simulink model "ltslqgservo"  (Simulink 8.0)
settings: Solver=ode1  StartTime=0.0  StopTime=stoptime  FixedStep=(1/10000)  RelTol=1e-3
values from neighbouring files (symbols this model uses):
  Ahat = Ap-Bp*Kpmcv    [main (ADMIN-PC's conflicted copy 2013-10-01).m]    (also in main.m = Ap-Bp*Kplqg)
  Ahat1 = Ayaw-Byaw*Kymcv    [main (ADMIN-PC's conflicted copy 2013-10-01).m]    (also in main.m = Ayaw-Byaw*Kylqg)
  Bhat = [Bp Gp]    [main (ADMIN-PC's conflicted copy 2013-10-01).m]    (also in main.m)
  Bhat1 = [Byaw Gyaw]    [main (ADMIN-PC's conflicted copy 2013-10-01).m]    (also in main.m)
  Chat = eye(4,4)    [main (ADMIN-PC's conflicted copy 2013-10-01).m]    (also in main.m)
  Chat1 = eye(4,4)    [main (ADMIN-PC's conflicted copy 2013-10-01).m]    (also in main.m)
  Dhat = zeros(4,2)    [main (ADMIN-PC's conflicted copy 2013-10-01).m]    (also in main.m)
  Dhat1 = zeros(4,2)    [main (ADMIN-PC's conflicted copy 2013-10-01).m]    (also in main.m)
  dt = 0.0001    [main (ADMIN-PC's conflicted copy 2013-10-01).m]    (also in main.m)
  Khat = Kpmcv    [main (ADMIN-PC's conflicted copy 2013-10-01).m]    (also in main.m = Kplqg)
  Khat1 = Kymcv    [main (ADMIN-PC's conflicted copy 2013-10-01).m]    (also in main.m = Kylqg)
undefined symbols (not defined in the file): clock, W
settings Model: Creator=Firdous  LastModifiedBy=salvatoregiorgi
settings DataIOCC: LimitDataPoints=off  SignalLoggingSaveFormat=ModelDataLogs  SaveState=on
settings DebuggingCC: FcnCallInpInsideContextMsg=EnableAllAsWarning
settings GRTTargetCC: CombineOutputUpdateFcns=off  GRTInterface=on

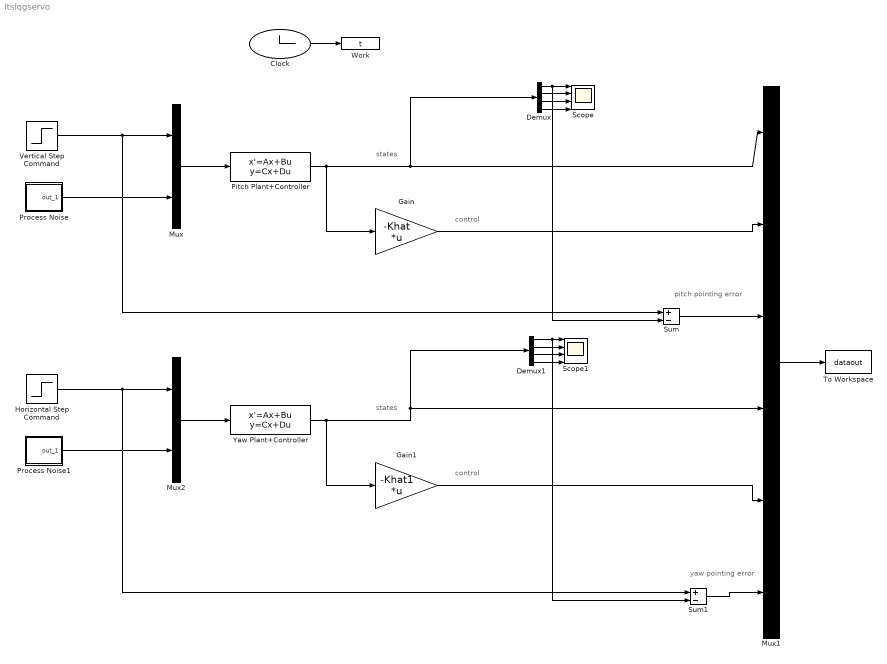
== system ltslqgservo ==
  note: states
  note: control
  note: states
  note: control
  note: pitch pointing error
  note: yaw pointing error
  Clock : Clock
  Demux : Demux
  Demux1 : Demux
  Gain : Gain  Gain=-Khat  Multiplication=Matrix(K*u)
  Gain1 : Gain  Gain=-Khat1  Multiplication=Matrix(K*u)
  Horizontal Step Command : Step  Time=0  After=15.15  SampleTime=0
  Mux : Mux  Inputs=2
  Mux1 : Mux  Inputs=6
  Mux2 : Mux  Inputs=2
  Pitch Plant+Controller : StateSpace  A=Ahat  B=Bhat  C=Chat  D=Dhat  X0=[2 0 0 0]
  Process Noise : Subsystem  mask(Continuous White Noise.){Cov=W, Ts=dt, seed=round(100*sum(clock))}
      mask prompts: Cov "Noise Variance:"; Ts "Sample Time:"
      mask help:
      | White noise for continuous (s-domain) systems.
      | Band-limited using zero-order-hold.
      mask Help: Implemented using white noise into Zero Order Hold block. For faster simulation set sample time to highest value possible but in accordance with the fastest dynamics of system.
      mask Display: plot(1:20,rand(size(1:20)))
  Process Noise1 : Subsystem  mask(Continuous White Noise.){Cov=W, Ts=dt, seed=round(100*sum(clock))}
      mask prompts: Cov "Noise Variance:"; Ts "Sample Time:"
      mask help:
      | White noise for continuous (s-domain) systems.
      | Band-limited using zero-order-hold.
      mask Help: Implemented using white noise into Zero Order Hold block. For faster simulation set sample time to highest value possible but in accordance with the fastest dynamics of system.
      mask Display: plot(1:20,rand(size(1:20)))
  Scope : Scope  NumInputPorts=4
      settings: YMin=-5~-5~-5~-5  YMax=5~5~5~5
  Scope1 : Scope  NumInputPorts=4
      settings: YMin=-5~-5~-5~-5  YMax=5~5~5~5
  Sum : Sum  Inputs=+-
  Sum1 : Sum  Inputs=+-
  To Workspace : ToWorkspace  VariableName=dataout  SampleTime=-1
  Vertical Step Command : Step  Time=0  After=15.15  SampleTime=0
  Work : ToWorkspace  VariableName=t
      settings: MaxDataPoints=stoptime
  Yaw Plant+Controller : StateSpace  A=Ahat1  B=Bhat1  C=Chat1  D=Dhat1  X0=[2 0 0 0]
  wires:
  Clock/1 -> Work/1
  Pitch Plant+Controller/1 -> Gain/1, Mux1/1, Demux/1
  Mux1/1 -> To Workspace/1
  Vertical Step Command/1 -> Mux/1, Sum/1
  Gain/1 -> Mux1/2
  Process Noise/1(out_1) -> Mux/2
  Mux/1 -> Pitch Plant+Controller/1
  Demux/1 -> Scope/1, Sum/2
  Demux/2 -> Scope/2
  Demux/3 -> Scope/3
  Demux/4 -> Scope/4
  Yaw Plant+Controller/1 -> Gain1/1, Demux1/1, Mux1/4
  Horizontal Step Command/1 -> Mux2/1, Sum1/1
  Process Noise1/1(out_1) -> Mux2/2
  Mux2/1 -> Yaw Plant+Controller/1
  Demux1/2 -> Scope1/2
  Demux1/3 -> Scope1/3
  Demux1/4 -> Scope1/4
  Demux1/1 -> Scope1/1, Sum1/2
  Gain1/1 -> Mux1/5
  Sum/1 -> Mux1/3
  Sum1/1 -> Mux1/6

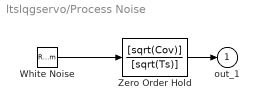
== system ltslqgservo/Process Noise ==
  White Noise : RandomNumber  Seed=seed  SampleTime=dt
  Zero Order Hold : DiscreteTransferFcn  Numerator=[sqrt(Cov)]  Denominator=[sqrt(Ts)]  SampleTime=Ts
  out_1 : Outport
  wires:
  Zero Order Hold/1 -> out_1/1
  White Noise/1 -> Zero Order Hold/1

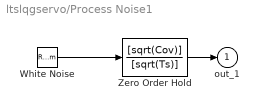
== system ltslqgservo/Process Noise1 ==
  White Noise : RandomNumber  Seed=seed  SampleTime=dt
  Zero Order Hold : DiscreteTransferFcn  Numerator=[sqrt(Cov)]  Denominator=[sqrt(Ts)]  SampleTime=Ts
  out_1 : Outport
  wires:
  Zero Order Hold/1 -> out_1/1
  White Noise/1 -> Zero Order Hold/1
